simulink model "ABS_SISO_SlipStateIOFBLModel"  (Simulink 7.1)
settings: Solver=ode45  StartTime=0.0  StopTime=3.4  RelTol=1e-3
undefined symbols (not defined in the file or in its folder): Bf, Cx, Fz, Im, l_0, Mt, mu_0, R0, v_initial, w_initial
settings Model: Creator=Nyandoro  LastModifiedBy=Nyandoro
settings OptimizationCC: InitFltsAndDblsToZero=off

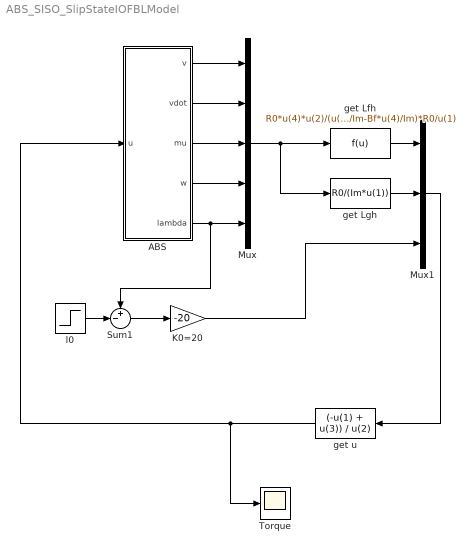
== system ABS_SISO_SlipStateIOFBLModel ==
  ABS : Subsystem
  K0=20 : Gain  Gain=-20  ParameterDataType=sfix(16)  ParameterScaling=2^0  OutDataType=sfix(16)  OutScaling=2^0
  Mux : Mux  Inputs=5
  Mux1 : Mux  Inputs=3
  Sum1 : Sum  Inputs=+-|  OutDataType=sfix(16)  OutScaling=2^0
  Torque : Scope
      settings: SaveName=ScopeData2
  get Lfh : Fcn  Expr=R0*u(4)*u(2)/(u(1)^2) - (u(3)*Fz*R0/Im-Bf*u(4)/Im)*R0/u(1)
  get Lgh : Fcn  Expr=R0/(Im*u(1))
  get u : Fcn  Orientation=left  Expr=(-u(1) + u(3)) / u(2)
  l0 : Step  Time=0  After=l_0  SampleTime=0
  wires:
  ABS/1(v) -> Mux/1
  ABS/2(vdot) -> Mux/2
  ABS/3(mu) -> Mux/3
  ABS/4(w) -> Mux/4
  Mux/1 -> get Lfh/1, get Lgh/1
  ABS/5(lambda) -> Mux/5, Sum1/1
  l0/1 -> Sum1/2
  Sum1/1 -> K0=20/1
  get Lfh/1 -> Mux1/1
  get Lgh/1 -> Mux1/2
  K0=20/1 -> Mux1/3
  Mux1/1 -> get u/1
  get u/1 -> ABS/1(u), Torque/1

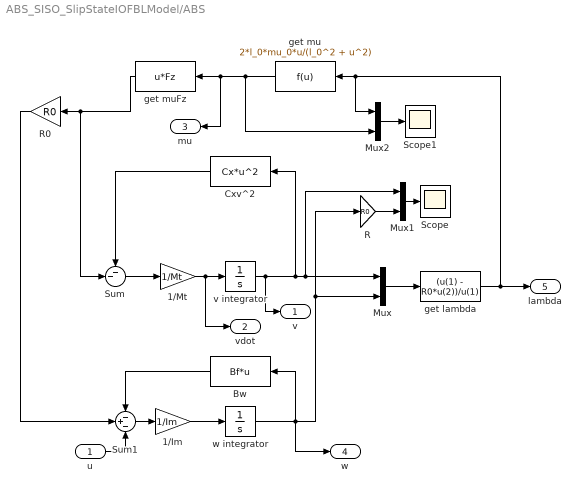
== system ABS_SISO_SlipStateIOFBLModel/ABS ==
  u : Inport
  1/Im : Gain  Gain=1/Im  ParameterDataType=sfix(16)  ParameterScaling=2^0  OutDataType=sfix(16)  OutScaling=2^0
  1/Mt : Gain  Gain=1/Mt  ParameterDataType=sfix(16)  ParameterScaling=2^0  OutDataType=sfix(16)  OutScaling=2^0
  Bw : Fcn  Orientation=left  Expr=Bf*u
  Cxv^2 : Fcn  Orientation=left  Expr=Cx*u^2
  Mux : Mux  Inputs=2
  Mux1 : Mux  Inputs=2
  Mux2 : Mux  Inputs=2
  R : Gain  Gain=R0  ParameterDataType=sfix(16)  ParameterScaling=2^0  OutDataType=sfix(16)  OutScaling=2^0
  R0 : Gain  Orientation=left  Gain=R0  ParameterDataType=sfix(16)  ParameterScaling=2^0  OutDataType=sfix(16)  OutScaling=2^0
  Scope : Scope
  Scope1 : Scope
  Sum : Sum  Inputs=--|  OutDataType=sfix(16)  OutScaling=2^0
  Sum1 : Sum  Inputs=-+-  OutDataType=sfix(16)  OutScaling=2^0
  get lambda : Fcn  Expr=(u(1) - R0*u(2))/u(1)
  get mu : Fcn  Orientation=left  Expr=2*l_0*mu_0*u/(l_0^2 + u^2)
  get muFz : Fcn  Orientation=left  Expr=u*Fz
  v integrator : Integrator  InitialCondition=v_initial
  w integrator : Integrator  InitialCondition=w_initial  LimitOutput=on  LowerSaturationLimit=0
  v : Outport  OutDataType=sfix(16)  OutScaling=2^0
  vdot : Outport  Port=2  OutDataType=sfix(16)  OutScaling=2^0
  mu : Outport  Orientation=left  Port=3  OutDataType=sfix(16)  OutScaling=2^0
  w : Outport  Port=4  OutDataType=sfix(16)  OutScaling=2^0
  lambda : Outport  Port=5  OutDataType=sfix(16)  OutScaling=2^0
  wires:
  v integrator/1 -> Cxv^2/1, Mux/1, Mux1/1, v/1
  Cxv^2/1 -> Sum/1
  1/Mt/1 -> v integrator/1, vdot/1
  Sum/1 -> 1/Mt/1
  w integrator/1 -> Bw/1, Mux/2, R/1, w/1
  Mux/1 -> get lambda/1
  get lambda/1 -> get mu/1, Mux2/1, lambda/1
  get mu/1 -> Mux2/2, mu/1, get muFz/1
  Sum1/1 -> 1/Im/1
  Bw/1 -> Sum1/1
  R0/1 -> Sum1/2
  1/Im/1 -> w integrator/1
  Mux1/1 -> Scope/1
  R/1 -> Mux1/2
  Mux2/1 -> Scope1/1
  u/1 -> Sum1/3
  get muFz/1 -> R0/1, Sum/2
